simulink model "Test"  (R2016b)
settings: Solver=ode5  StartTime=0.0  StopTime=100.0  FixedStep=0.01  RelTol=1e-3
settings Model: Creator=davide  LastModifiedBy=davide

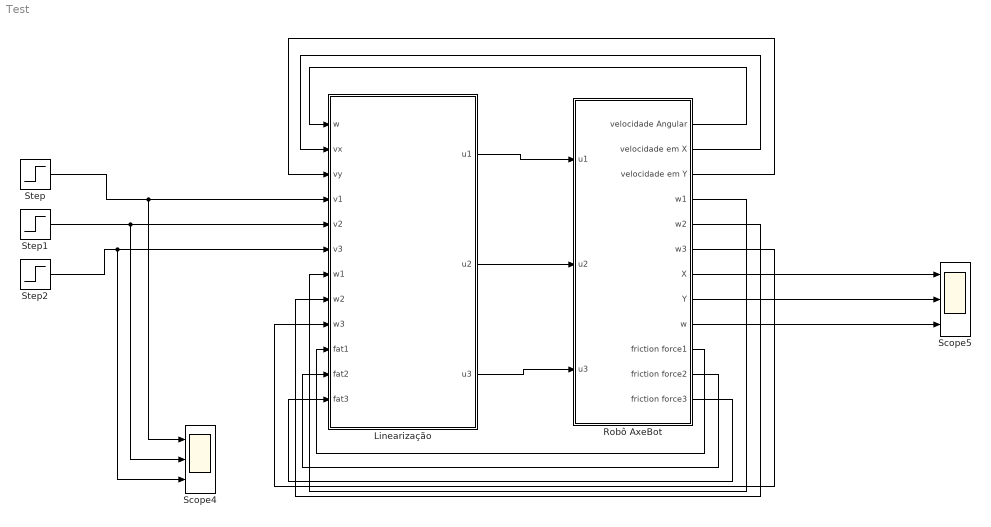
== system Test ==
  Linearização : MATLAB Function  TreatAsAtomicUnit=on
  Robô AxeBot : Subsystem
  Scope4 : Scope  NumInputPorts=3
  Scope5 : Scope  NumInputPorts=3
  Step : Step  SampleTime=0
  Step1 : Step  SampleTime=0
  Step2 : Step  SampleTime=0
  wires:
  Linearização/1(u1) -> Robô AxeBot/1(u1)
  Linearização/2(u2) -> Robô AxeBot/2(u2)
  Linearização/3(u3) -> Robô AxeBot/3(u3)
  Step1/1 -> Scope4/2, Linearização/5(v2)
  Step/1 -> Scope4/1, Linearização/4(v1)
  Step2/1 -> Scope4/3, Linearização/6(v3)
  Robô AxeBot/10(friction force1) -> Linearização/10(fat1)
  Robô AxeBot/11(friction force2) -> Linearização/11(fat2)
  Robô AxeBot/12(friction force3) -> Linearização/12(fat3)
  Robô AxeBot/8(Y) -> Scope5/2
  Robô AxeBot/7(X) -> Scope5/1
  Robô AxeBot/9(w) -> Scope5/3
  Robô AxeBot/1(velocidade Angular) -> Linearização/1(w)
  Robô AxeBot/2(velocidade em X) -> Linearização/2(vx)
  Robô AxeBot/3(velocidade em Y) -> Linearização/3(vy)
  Robô AxeBot/4(w1) -> Linearização/7(w1)
  Robô AxeBot/5(w2) -> Linearização/8(w2)
  Robô AxeBot/6(w3) -> Linearização/9(w3)

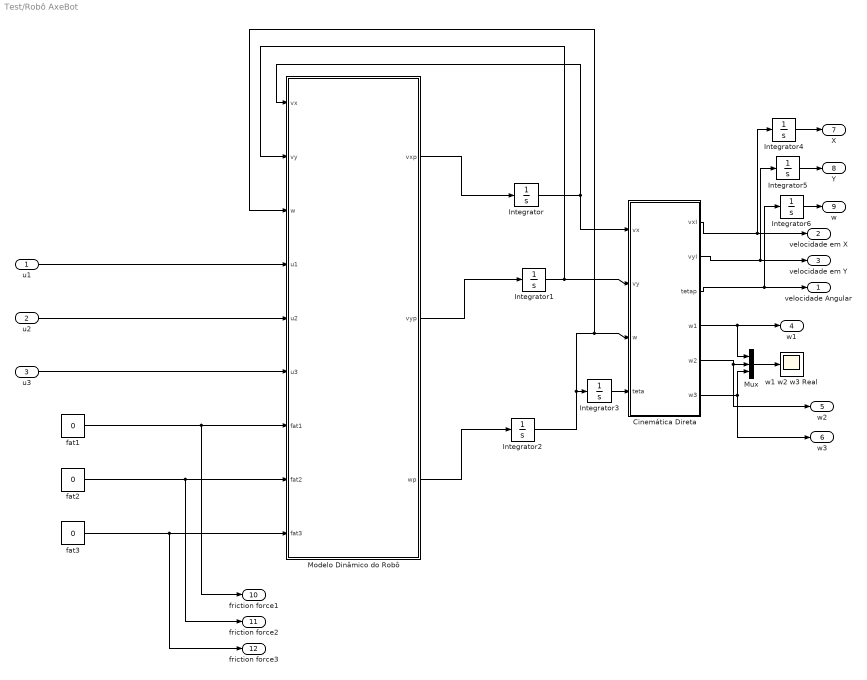
== system Test/Robô AxeBot ==
  u1 : Inport
  u2 : Inport  Port=2
  u3 : Inport  Port=3
  Cinemática Direta : MATLAB Function  TreatAsAtomicUnit=on
  Integrator{,1..6} (7 alike) : Integrator
  Modelo Dinâmico do Robô : MATLAB Function  TreatAsAtomicUnit=on
  Mux : Mux  Inputs=3
  fat1 : Constant  Value=0
  fat2 : Constant  Value=0
  fat3 : Constant  Value=0
  w1 w2 w3 Real : Scope
  velocidade Angular : Outport
  velocidade em X : Outport  Port=2
  velocidade em Y : Outport  Port=3
  w1 : Outport  Port=4
  w2 : Outport  Port=5
  w3 : Outport  Port=6
  X : Outport  Port=7
  Y : Outport  Port=8
  w : Outport  Port=9
  friction force1 : Outport  Port=10
  friction force2 : Outport  Port=11
  friction force3 : Outport  Port=12
  wires:
  Cinemática Direta/3(tetap) -> velocidade Angular/1, Integrator6/1
  Cinemática Direta/1(vxI) -> velocidade em X/1, Integrator4/1
  Cinemática Direta/2(vyI) -> velocidade em Y/1, Integrator5/1
  Modelo Dinâmico do Robô/3(wp) -> Integrator2/1
  Integrator2/1 -> Cinemática Direta/3(w), Modelo Dinâmico do Robô/3(w), Integrator3/1
  Integrator1/1 -> Modelo Dinâmico do Robô/2(vy), Cinemática Direta/2(vy)
  Modelo Dinâmico do Robô/2(vyp) -> Integrator1/1
  Modelo Dinâmico do Robô/1(vxp) -> Integrator/1
  Integrator/1 -> Cinemática Direta/1(vx), Modelo Dinâmico do Robô/1(vx)
  Mux/1 -> w1 w2 w3 Real/1
  Cinemática Direta/4(w1) -> Mux/1, w1/1
  Cinemática Direta/5(w2) -> Mux/2, w2/1
  Cinemática Direta/6(w3) -> Mux/3, w3/1
  Integrator3/1 -> Cinemática Direta/4(teta)
  Integrator4/1 -> X/1
  Integrator5/1 -> Y/1
  Integrator6/1 -> w/1
  fat1/1 -> friction force1/1, Modelo Dinâmico do Robô/7(fat1)
  fat2/1 -> friction force2/1, Modelo Dinâmico do Robô/8(fat2)
  fat3/1 -> friction force3/1, Modelo Dinâmico do Robô/9(fat3)
  u3/1 -> Modelo Dinâmico do Robô/6(u3)
  u2/1 -> Modelo Dinâmico do Robô/5(u2)
  u1/1 -> Modelo Dinâmico do Robô/4(u1)

== matlab function Test/Robô AxeBot/Modelo Dinâmico do Robô ==
  settings: fimath=|
      | fimath(...
      | 'RoundMode', 'floor',...
      | 'OverflowMode', 'wrap',...
      | 'ProductMode', 'KeepLSB', 'ProductWordLength', 32,...
      | 'SumMode', 'KeepLSB', 'SumWordLength', 32,...
      | 'CastBeforeSum', false)
  data: vx input; vxp output; vy input; w input; u1 input; u2 input; u3 input; vyp output; wp output; fat1 input; fat2 input; fat3 input
function [vxp,vyp,wp] = MDRobo(vx,vy,w,u1,u2,u3,fat1,fat2,fat3)

N=19; %Fator de redução de velocidade (admensional)
eta=0.83; %Eficiencia mecanica do acoplamento (admensional)
kt=0.0059; %Constante de torque Nm/A
kem=0.0059;  %Constante de força contra-eletromotriz Volt s/rad
Jm=3.88e-7; % Inercia do atuador 3 em Kilogramos-metros^2 kgm^2
J=2.125; % Inercia da base movel em Kilogramos-metros^2 kgm^2
l=0.09; %Distancia do centro da base móvel ao centro da roda 3 metros m
rw=0.072; %Raio de cada roda 3 metros m
M=1.830; %Massa da base móvel em Kilogramos Kg
R=1.710; %Resistencia de cada armadura Ohm
bo = 2.4e-6;
vxp=0;
vyp=0;
wp=0;
H = [1/M 0 0; 0 1/M 0; 0 0 1/J];
B = [0 cos(pi/6) -cos(pi/6); -1 sin(pi/6) sin(pi/6); l l l];
I = [1 0 0; 0 1 0; 0 0 1];
G = I+(H*B*B.'*((((eta*N)^2)*Jm)/(rw^2)));



Gi=inv(G);

A= (-(Gi*H*B*B.'*(((kt*kem)/R)+bo).*(((eta*N)^2)/(rw^2))*[vx;vy;w])+Gi*H*B*((kt*eta*N)/(rw*R))*[u1;u2;u3])-Gi*H*B*[fat1;fat2;fat3];
vxp=A(1,:);
vyp=A(2,:);
wp=A(3,:);

== matlab function Test/Robô AxeBot/Cinemática Direta ==
  settings: fimath=|
      | fimath(...
      | 'RoundMode', 'floor',...
      | 'OverflowMode', 'wrap',...
      | 'ProductMode', 'KeepLSB', 'ProductWordLength', 32,...
      | 'SumMode', 'KeepLSB', 'SumWordLength', 32,...
      | 'CastBeforeSum', false)
  data: vx input; vxI output; vy input; vyI output; w input; tetap output; teta input; w1 output; w2 output; w3 output
function [vxI,vyI,tetap,w1,w2,w3] = CD(vx,vy,w,teta)
% This block supports an embeddable subset of the MATLAB language.
% See the help menu for details.
N=19; %Fator de redução de velocidade (admensional)
eta=0.83; %Eficiencia mecanica do acoplamento (admensional)
l=0.09; %Distancia do centro da base móvel ao centro da roda 3 metros m
rw=0.072; %Raio de cada roda 3 metros m
B = [0 cos(pi/6) -cos(pi/6); -1 sin(pi/6) sin(pi/6); l l l];


T=[cos(teta) -sin(teta) 0; sin(teta) cos(teta) 0; 0 0 1]*[vx;vy;w];

vxI=T(1,:);
vyI=T(2,:);
tetap=T(3,:);

W=((eta*N)/rw)*B'*[vx;vy;w];

w1=W(1,:);
w2=W(2,:);
w3=W(3,:);

== matlab function Test/Linearização ==
  settings: fimath=|
      | fimath(...
      | 'RoundMode', 'floor',...
      | 'OverflowMode', 'wrap',...
      | 'ProductMode', 'KeepLSB', 'ProductWordLength', 32,...
      | 'SumMode', 'KeepLSB', 'SumWordLength', 32,...
      | 'CastBeforeSum', false)
  data: w input; vx input; vy input; v1 input; v2 input; v3 input; w1 input; w2 input; w3 input; u1 output; u2 output; u3 output; fat1 input; fat2 input; fat3 input
function [u1,u2,u3] = LinearizacaoEE(w,vx,vy,v1,v2,v3,w1,w2,w3,fat1,fat2,fat3)

N=19; %Fator de redução de velocidade (admensional)
eta=0.83; %Eficiencia mecanica do acoplamento (admensional)
kt=0.0059; %Constante de torque Nm/A
kem=0.0059;  %Constante de força contra-eletromotriz Volt s/rad
Jm=3.88e-7; % Inercia do atuador 3 em Kilogramos-metros^2 kgm^2
J=2.125; % Inercia da base movel em Kilogramos-metros^2 kgm^2
l=0.09; %Distancia do centro da base móvel ao centro da roda 3 metros m
rw=0.072; %Raio de cada roda 3 metros m
M=1.830; %Massa da base móvel em Kilogramos Kg
R=1.710; %Resistencia de cada armadura Ohm
bo = 2.4e-6;

vxp=0;
vyp=0;
wp=0;

H = [1/M 0 0; 0 1/M 0; 0 0 1/J];
B = [0 cos(pi/6) -cos(pi/6); -1 sin(pi/6) sin(pi/6); l l l];
I = [1 0 0; 0 1 0; 0 0 1];
G = I+(H*B*B.'*((((eta*N)^2)*Jm)/(rw^2)));

Gi=inv(G);
Ai=((eta*N)/rw)*B.';
Gx=(Ai*Gi*H*B)*((kt*eta*N)/(R*rw));
GxI=inv(Gx);

U=GxI*(Ai*Gi*H*B*[fat1;fat2;fat3]+(Ai*Gi*H*B*((kt*kem/R)+bo)*((eta*N)/rw)*[w1;w2;w3]))+GxI*[v1;v2;v3];

u1=U(1,:);
u2=U(2,:);
u3=U(3,:);
